simulink model "dev_sim_lineal_lqr"  (R2019b)
settings: Solver=VariableStepAuto  StartTime=0.0  StopTime=100.0  RelTol=1e-3
values from neighbouring files (symbols this model uses):
  A_0 = eval(A_0)    [modelo.m]    (also in modelo_var.m; parametros.mat = [0 -3.26931291643 0 0.71460251427 0 0 0 0 1 -0.0325743287495)
  B_0 = eval(B_0)    [modelo.m]    (also in modelo_var.m; parametros.mat = [0 0 0 0 0 0 1190.47619048 0 0 0 0 0 ... (16 elements, 8x2)])
  C_0 = eval(C_0)    [modelo.m]    (also in modelo_var.m; parametros.mat = [1 0 0 0 0 1 0 0 0 0 0 0 ... (16 elements, 2x8)])
  D_0 = eval(D_0)    [modelo.m]    (also in modelo_var.m; parametros.mat = [0  0; 0  0])
undefined symbols (not defined in the file or in its folder): K
settings Model: Creator=tronc  LastModifiedBy=tronc

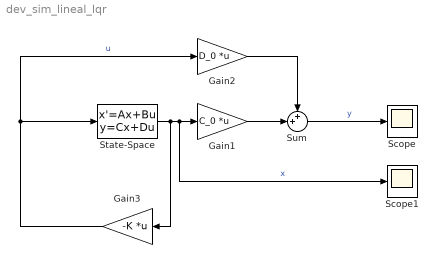
== system dev_sim_lineal_lqr ==
  Gain1 : Gain  Gain=C_0  Multiplication=Matrix(K*u)
  Gain2 : Gain  Gain=D_0  Multiplication=Matrix(K*u)
  Gain3 : Gain  Gain=-K  Multiplication=Matrix(K*u)
  Scope : Scope
  Scope1 : Scope
  State-Space : StateSpace  A=A_0  B=B_0  C=eye(8)  D=zeros(8,2)  InitialCondition=[1 1 0 0 0 0 0 0]
  Sum : Sum  Inputs=++|
  wires:
  State-Space/1 -> Gain3/1, Scope1/1, Gain1/1  "x"
  Gain3/1 -> Gain2/1, State-Space/1  "u"
  Sum/1 -> Scope/1  "y"
  Gain2/1 -> Sum/1
  Gain1/1 -> Sum/2
